simulink model "blink_challenge_sf"  (Simulink 7.1)
settings: Solver=FixedStepDiscrete  StartTime=0.0  StopTime=60.0  FixedStep=0.1  RelTol=1e-3
libraries: arduino_io_lib x9
settings Model: Creator=gvallabh  LastModifiedBy=gcampa
settings OptimizationCC: InitFltsAndDblsToZero=off
settings DebuggingCC: StrictBusMsg=ErrorLevel1
settings HardwareCC: ProdBitPerInt=16  ProdIntDivRoundTo=Zero  ProdEndianess=LittleEndian  ProdWordSize=8  ProdHWDeviceType=Atmel->AVR  TargetIntDivRoundTo=Zero  TargetEndianess=LittleEndian  TargetHWDeviceType=MATLAB Host  ProdEqTarget=off
settings RTWCC: SystemTargetFile=rsim.tlc  TemplateMakefile=rsim_default_tmf  Description=Rapid Simulation Target  ProcessScript=rsim_make_rtw_hook
settings RSimTargetCC: TargetFunctionLibrary=ANSI_C  IsPILTarget=off  EnableShiftOperators=on  PortableWordSizes=off

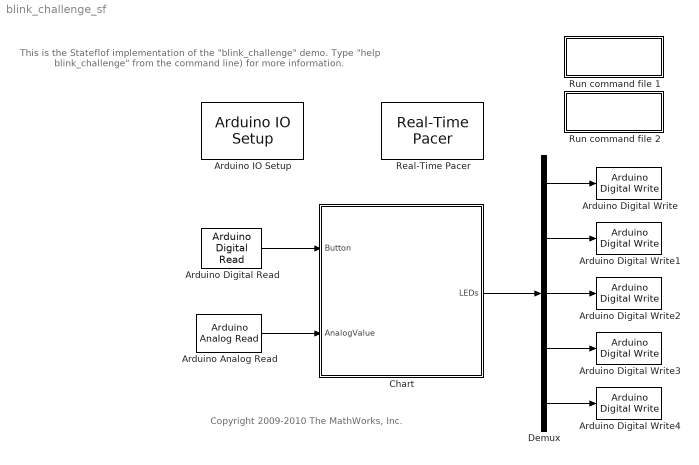
== system blink_challenge_sf ==
  note: Copyright 2009-2010 The MathWorks, Inc.
  note: This is the Stateflof implementation of the "blink_challenge"
      | demo. Type "help blink_challenge" from the command line)
      | for more information.
  Arduino Analog Read : arduino_io_lib/Arduino Analog Read  arduinoVar=Temporary arduino variable: Arduino1  arduinoPin=2  T=0.1
  Arduino Digital Read : arduino_io_lib/Arduino Digital Read  arduinoVar=Temporary arduino variable: Arduino1  arduinoPin=2  T=0.1
  Arduino Digital Write : arduino_io_lib/Arduino Digital Write  arduinoVar=Temporary arduino variable: Arduino1  arduinoPin=9  T=0.1
  Arduino Digital Write1 : arduino_io_lib/Arduino Digital Write  arduinoVar=Temporary arduino variable: Arduino1  arduinoPin=10  T=0.1
  Arduino Digital Write2 : arduino_io_lib/Arduino Digital Write  arduinoVar=Temporary arduino variable: Arduino1  arduinoPin=11  T=0.1
  Arduino Digital Write3 : arduino_io_lib/Arduino Digital Write  arduinoVar=Temporary arduino variable: Arduino1  arduinoPin=12  T=0.1
  Arduino Digital Write4 : arduino_io_lib/Arduino Digital Write  arduinoVar=Temporary arduino variable: Arduino1  arduinoPin=13  T=0.1
  Arduino IO Setup : arduino_io_lib/Arduino IO Setup  Priority=3  arduinoVar=Temporary arduino variable: Arduino1  comPort=COM9
  Chart : Stateflow chart  TreatAsAtomicUnit=on
      settings: PermitHierarchicalResolution=ParametersOnly
  Demux : Demux  Outputs=ones(5,1)
  Real-Time Pacer : arduino_io_lib/Real-Time Pacer  simTimePerRealTime=1
  Run command file 1 : Subsystem
      settings: OpenFcn=blink_challenge_sim
      mask Display: disp('Simulink \nImplementation')
  Run command file 2 : Subsystem
      settings: OpenFcn=edit('blink_challenge.m');
      mask Display: disp('MATLAB \nImplementation')
  wires:
  Arduino Digital Read/1 -> Chart/1(Button)
  Arduino Analog Read/1 -> Chart/2(AnalogValue)
  Chart/1(LEDs) -> Demux/1
  Demux/1 -> Arduino Digital Write/1
  Demux/2 -> Arduino Digital Write1/1
  Demux/3 -> Arduino Digital Write2/1
  Demux/4 -> Arduino Digital Write3/1
  Demux/5 -> Arduino Digital Write4/1

== system blink_challenge_sf/Run command file 1 ==

== system blink_challenge_sf/Run command file 2 ==

== stateflow chart Chart ==
  state SelectMode [parallel]
    settings: executionOrder=1
    state ButtonPressed
    state ButtonReleased
      entry: send(ChangeMode)
    ButtonPressed -> ButtonReleased : [Button == 0]
    ButtonReleased -> ButtonPressed : [Button == 1]
    (default) -> ButtonPressed
  state ExecuteMode [parallel]
    during: NumTicks = RawValueToTicks(AnalogValue);
    settings: executionOrder=2
    state All_LEDs_Off
      entry, during: LEDs = 0;
    state All_LEDs_On
      entry, during: LEDs = 1;
    state All_LEDs_Blink
      state LEDS_On
        entry: LEDs = 1;
      state LEDs_Off
        entry: LEDs = 0;
      LEDS_On -> LEDs_Off : after(NumTicks,tick)
      LEDs_Off -> LEDS_On : after(NumTicks,tick)
      (default) -> LEDS_On
    state All_LEDs_Cycle
      entry: index = 0; LEDs = 0;
      state Set_one_LED
        entry:
        setLEDs(index);
        index = (index + 1) %% 5;
      Set_one_LED -> (junction 16) : after(NumTicks,tick)
      (junction 16) -> Set_one_LED
    All_LEDs_Off -> All_LEDs_On : ChangeMode
    (default) -> All_LEDs_Off
    All_LEDs_On -> All_LEDs_Blink : ChangeMode
    All_LEDs_Blink -> All_LEDs_Cycle : ChangeMode
    All_LEDs_Cycle -> All_LEDs_Off : ChangeMode
  data: index local double size=[1 1]; analogValue function_input double; numTicks function_output double; ledIndex function_input double; Button input double; AnalogValue input double; LEDs output uint8 size=[5 1]; NumTicks local double
  events: ChangeMode local EITHER_EDGE_EVENT
  function numTicks = RawValueToTicks(analogValue):
    | function numTicks = RawValueToTicks(analogValue)
    | maxAnalogValue = 1024;
    | sampleTime = 0.1; 
    | normalizedValue = 0.5 * (analogValue / maxAnalogValue);
    | numTicks = ceil(normalizedValue / sampleTime);
  function setLEDs(ledIndex):
    | function setLEDs(ledIndex)
    | 
    | % ledIndex is zero-based
    | LEDs = zeros(5,1, 'uint8');
    | LEDs(ledIndex+1) = 1;
